simulink model "smd"  (Simulink 10.2)
settings: Solver=ode45  StartTime=0.0  StopTime=10.0  RelTol=1e-3  EnableMultiTasking=on
undefined symbols (not defined in the file or in its folder): b, k, m
settings Model: Creator=Chris Jobling  LastModifiedBy=eechris
settings DataIOCC: LimitDataPoints=on
settings OptimizationCC: ExpressionDepthLimit=2147483647
settings DebuggingCC: SolverPrmCheckMsg=warning  StateNameClashWarn=warning

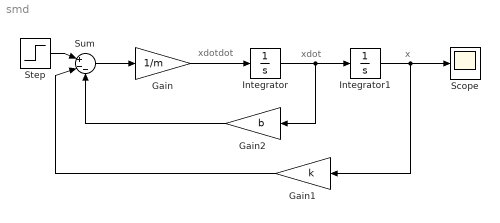
== system smd ==
  note: xdot
  note: xdotdot
  note: x
  Gain : Gain  Gain=1/m
  Gain1 : Gain  Gain=k
  Gain2 : Gain  Gain=b
  Integrator : Integrator
  Integrator1 : Integrator
  Scope : Scope
  Step : Step  SampleTime=0
  Sum : Sum  Inputs=|+--
  wires:
  Integrator/1 -> Integrator1/1, Gain2/1
  Gain/1 -> Integrator/1
  Integrator1/1 -> Scope/1, Gain1/1
  Gain2/1 -> Sum/3
  Gain1/1 -> Sum/2
  Step/1 -> Sum/1
  Sum/1 -> Gain/1
